simulink library "Power_Shaft4_Ideal_L1_R1_L2_R2"  (R2022b)
settings: Solver=VariableStepAuto  StartTime=0.0  StopTime=10.0  RelTol=1e-3
undefined symbols (not defined in the file or in its folder): ShaftL1, ShaftL2, ShaftR1, ShaftR2
libraries: fl_lib x5, Power_Components x4, nesl_utility x4, sm_lib x1
Description:
  | Component of Simscape Vehicle Templates Library
  | 
  | Copyright 2018-2024 The MathWorks, Inc.
settings Model: Creator=smiller  LastModifiedBy=smiller
settings SolverCC: AlgebraicLoopSolver=TrustRegion
settings DataIOCC: ReturnWorkspaceOutputs=off
settings DebuggingCC: UnconnectedInputMsg=warning  UnconnectedOutputMsg=warning  UnconnectedLineMsg=warning  SFMachineParentedDataDiag=warning  ArithmeticOperatorsInVariantConditions=warning
settings ModelReferenceCC: EnableRefExpFcnMdlSchedulingChecks=on
settings SFSimCC: CustomCodeUndefinedFunction=UseInterfaceOnly
settings RTWCC: DLArmComputeVersion=19.05

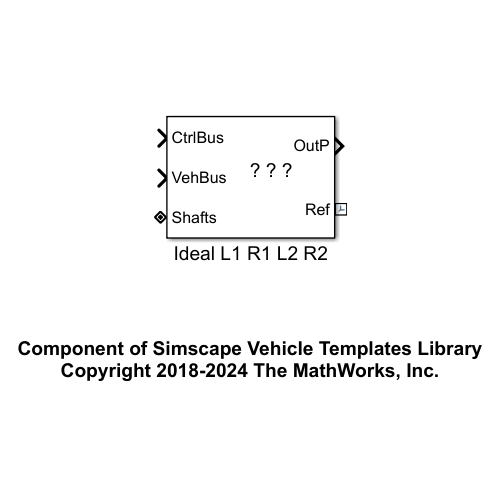
[thumbnail: Simulink's stored preview of the top-level diagram]
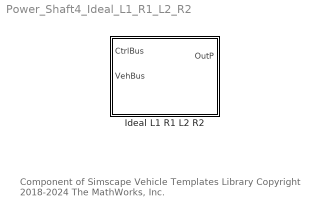
== system Power_Shaft4_Ideal_L1_R1_L2_R2 ==
  note: Component of Simscape Vehicle Templates Library
      | Copyright 2018-2024 The MathWorks, Inc.
  Ideal L1 R1 L2 R2 : Subsystem  mask(Four Ideal Motors, Wheels L1, L2, R1, R2){motor_ts_l1=100, motor_ts_r1=100, motor_ts_l2=100, motor_ts_r2=100}
      mask prompts: motor_ts_l1 "Wheel L1 Motor Cutoff Frequency (Hz)"; motor_ts_r1 "Wheel R1 Motor Cutoff Frequency (Hz)"; motor_ts_l2 "Wheel L2 Motor Cutoff Frequency (Hz)"; motor_ts_r2 "Wheel R2 Motor Cutoff Frequency (Hz)"
      mask help: Models four ideal motors connected to the four driveshafts in vehicle driveline.
      mask Display: image('sm_car_vehicle_power_i4motor_IMAGE.png');

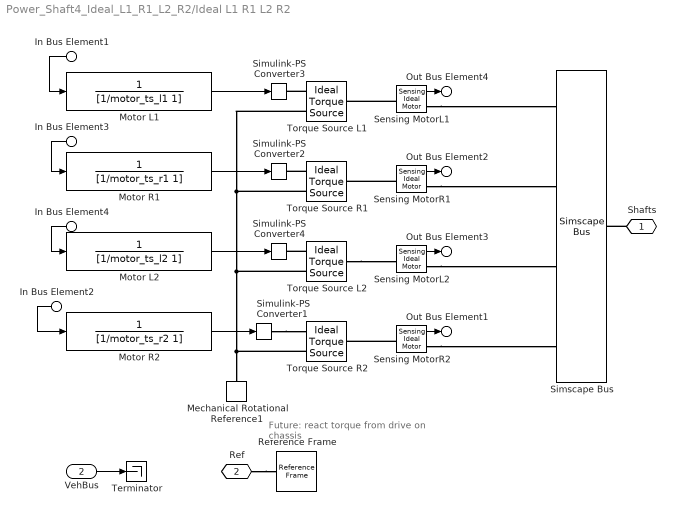
== system Power_Shaft4_Ideal_L1_R1_L2_R2/Ideal L1 R1 L2 R2 ==
  note: Future: react torque from
      | drive on chassis
  In Bus Element1 : Inport  PortName=CtrlBus  Element=MMotorL1Demand
  In Bus Element2 : Inport  PortName=CtrlBus  Element=MMotorR2Demand
  In Bus Element3 : Inport  PortName=CtrlBus  Element=MMotorR1Demand
  In Bus Element4 : Inport  PortName=CtrlBus  Element=MMotorL2Demand
  VehBus : Inport  Port=2
  Mechanical Rotational Reference1 : fl_lib/Mechanical/Rotational Elements/Mechanical Rotational Reference
  Motor L1 : TransferFcn  Denominator=[1/motor_ts_l1 1]
  Motor L2 : TransferFcn  Denominator=[1/motor_ts_l2 1]
  Motor R1 : TransferFcn  Denominator=[1/motor_ts_r1 1]
  Motor R2 : TransferFcn  Denominator=[1/motor_ts_r2 1]
  Reference Frame : sm_lib/Frames and Transforms/Reference Frame
  Sensing MotorL1 : Power_Components/Sensing Ideal Motor  SystemSampleTime=-1  VariantActivationTime=update diagram  Latency=0  AutoFrameSizeCalculation=off
  Sensing MotorL2 : Power_Components/Sensing Ideal Motor  SystemSampleTime=-1  VariantActivationTime=update diagram  Latency=0  AutoFrameSizeCalculation=off
  Sensing MotorR1 : Power_Components/Sensing Ideal Motor  SystemSampleTime=-1  VariantActivationTime=update diagram  Latency=0  AutoFrameSizeCalculation=off
  Sensing MotorR2 : Power_Components/Sensing Ideal Motor  SystemSampleTime=-1  VariantActivationTime=update diagram  Latency=0  AutoFrameSizeCalculation=off
  Simscape Bus : SimscapeBus  HierarchyStrings=ShaftL1;ShaftR1;ShaftL2;ShaftR2
  Simulink-PS Converter{1..4} (4 alike) : nesl_utility/Simulink-PS Converter  PhysicalDomain=network_engine_domain  SubClassName=ps_input  LeftPortType=input  RightPortType=output  PseudoPeriodic=off  Frequencies=[]  NoiseDistribution=none  NoiseParameters=[]  Unit=1  AffineConversion=off  FilteringAndDerivatives=provide  SimscapeFilterOrder=1  InputFilterTimeConstant=0.001  UdotUserProvided=0
  Terminator : Terminator
  Torque Source L1 : fl_lib/Mechanical/Mechanical Sources/Ideal Torque Source
  Torque Source L2 : fl_lib/Mechanical/Mechanical Sources/Ideal Torque Source
  Torque Source R1 : fl_lib/Mechanical/Mechanical Sources/Ideal Torque Source
  Torque Source R2 : fl_lib/Mechanical/Mechanical Sources/Ideal Torque Source
  Shafts : PMIOPort  Side=Left
  Ref : PMIOPort  Port=2  Side=Right
  Out Bus Element4 : Outport  VectorParamsAs1DForOutWhenUnconnected=off  PortName=OutP  Element=MotorL1
  Out Bus Element2 : Outport  VectorParamsAs1DForOutWhenUnconnected=off  PortName=OutP  Element=MotorR1
  Out Bus Element3 : Outport  VectorParamsAs1DForOutWhenUnconnected=off  PortName=OutP  Element=MotorL2
  Out Bus Element1 : Outport  VectorParamsAs1DForOutWhenUnconnected=off  PortName=OutP  Element=MotorR2
  wires:
  In Bus Element1/1 -> Motor L1/1
  VehBus/1 -> Terminator/1
  In Bus Element2/1 -> Motor R2/1
  Sensing MotorL1/1 -> Out Bus Element4/1
  Motor L1/1 -> Simulink-PS Converter3/1
  Motor R2/1 -> Simulink-PS Converter1/1
  Motor R1/1 -> Simulink-PS Converter2/1
  In Bus Element3/1 -> Motor R1/1
  In Bus Element4/1 -> Motor L2/1
  Motor L2/1 -> Simulink-PS Converter4/1
  Sensing MotorR1/1 -> Out Bus Element2/1
  Sensing MotorL2/1 -> Out Bus Element3/1
  Sensing MotorR2/1 -> Out Bus Element1/1
  connections:
  Sensing MotorR2/LConn1 -- Torque Source R2/LConn1
  Sensing MotorL1/LConn1 -- Torque Source L1/LConn1
  Torque Source L1/RConn2 -- Torque Source R1/RConn2 -- Torque Source L2/RConn2 -- Torque Source R2/RConn2 -- Mechanical Rotational Reference1/LConn1
  Shafts/RConn1 -- Simscape Bus/RConn1
  Ref/RConn1 -- Reference Frame/RConn1
  Torque Source L1/RConn1 -- Simulink-PS Converter3/RConn1
  Sensing MotorR2/RConn1 -- Simscape Bus/LConn4
  Simulink-PS Converter1/RConn1 -- Torque Source R2/RConn1
  Sensing MotorL1/RConn1 -- Simscape Bus/LConn1
  Sensing MotorR1/LConn1 -- Torque Source R1/LConn1
  Sensing MotorR1/RConn1 -- Simscape Bus/LConn2
  Torque Source R1/RConn1 -- Simulink-PS Converter2/RConn1
  Torque Source L2/LConn1 -- Sensing MotorL2/LConn1
  Sensing MotorL2/RConn1 -- Simscape Bus/LConn3
  Torque Source L2/RConn1 -- Simulink-PS Converter4/RConn1
